simulink model "fusionAlg"  (R2018b)
settings: Solver=FixedStepDiscrete  StartTime=0.0  StopTime=inf  FixedStep=0.01  RelTol=1e-3
PostLoadFcn:
  | if any(exist('dsrtsu_mdlpostloadfcn', 'file') ~= 0), dsrtsu_mdlpostloadfcn('Execute', bdroot); end
model workspace (MAT data in the model file):
  handle : class17 (value not decoded)
(part 2 of 24)

== system fusionAlg/FUSION /FUS_DataAdapter/RadarAdapter/Subsystem15 ==
  <x67_37_Obj_23> : Inport
  Bus Creator : BusCreator  Inputs=2  OutDataTypeStr=Bus: FUS_UINT8_RESERVED_ST
      settings: InheritFromInputs=off
  Bus Creator1 : BusCreator  Inputs=17  OutDataTypeStr=Bus: FUS_RADAR_OBJ_ST  NonVirtualBus=on
      settings: InheritFromInputs=off
  Bus Selector1 : BusSelector  OutputSignals=Obj_ObstacleProb,Obj_XPos_Stdev,Obj_YPos_Stdev,Obj_XVelRel_Stdev,Obj_XAccRel,Obj_ExstProb,Obj_YVelRel,Obj_XVelRel,Obj_XPos,Obj_YPos,Obj_ID,Obj_UpdateFlag,Obj_ValidFlag,Obj_MotionPattern,Obj_Type,Obj_MeasFlag
  Constant : Constant  Value=0  OutDataTypeStr=uint8
  Constant1 : Constant  Value=0  OutDataTypeStr=uint8
  Data Type Conversion : DataTypeConversion  OutDataTypeStr=uint16
  Data Type Conversion{1..5} (5 alike) : DataTypeConversion  OutDataTypeStr=uint8
  <OBJ_23> : Outport
  wires:
  Bus Selector1/10 -> Bus Creator1/10  "<Obj_YPos>"
  Constant1/1 -> Bus Creator/2
  Bus Selector1/8 -> Bus Creator1/8  "<Obj_XVelRel>"
  Bus Selector1/14 -> Data Type Conversion3/1  "<Obj_MotionPattern>"
  Bus Creator1/1 -> <OBJ_23>/1
  Bus Selector1/11 -> Data Type Conversion/1  "<Obj_ID>"
  Bus Selector1/16 -> Data Type Conversion5/1  "<Obj_MeasFlag>"
  Bus Selector1/2 -> Bus Creator1/2  "<Obj_XPos_Stdev>"
  Bus Selector1/6 -> Bus Creator1/6  "<Obj_ExstProb>"
  Bus Selector1/1 -> Bus Creator1/1  "<Obj_ObstacleProb>"
  Bus Selector1/15 -> Data Type Conversion4/1  "<Obj_Type>"
  Constant/1 -> Bus Creator/1
  Bus Selector1/13 -> Data Type Conversion2/1  "<Obj_ValidFlag>"
  Bus Selector1/9 -> Bus Creator1/9  "<Obj_XPos>"
  Bus Selector1/4 -> Bus Creator1/4  "<Obj_XVelRel_Stdev>"
  Bus Selector1/3 -> Bus Creator1/3  "<Obj_YPos_Stdev>"
  Bus Selector1/5 -> Bus Creator1/5  "<Obj_XAccRel>"
  Bus Selector1/7 -> Bus Creator1/7  "<Obj_YVelRel>"
  Bus Selector1/12 -> Data Type Conversion1/1  "<Obj_UpdateFlag>"
  <x67_37_Obj_23>/1 -> Bus Selector1/1
  Bus Creator/1 -> Bus Creator1/17
  Data Type Conversion/1 -> Bus Creator1/11
  Data Type Conversion1/1 -> Bus Creator1/12
  Data Type Conversion2/1 -> Bus Creator1/13
  Data Type Conversion3/1 -> Bus Creator1/14
  Data Type Conversion4/1 -> Bus Creator1/15
  Data Type Conversion5/1 -> Bus Creator1/16

== system fusionAlg/FUSION /FUS_DataAdapter/RadarAdapter/Subsystem16 ==
  <x5E_2E_Obj_14> : Inport
  Bus Creator : BusCreator  Inputs=2  OutDataTypeStr=Bus: FUS_UINT8_RESERVED_ST
      settings: InheritFromInputs=off
  Bus Creator1 : BusCreator  Inputs=17  OutDataTypeStr=Bus: FUS_RADAR_OBJ_ST  NonVirtualBus=on
      settings: InheritFromInputs=off
  Bus Selector1 : BusSelector  OutputSignals=Obj_ObstacleProb,Obj_XPos_Stdev,Obj_YPos_Stdev,Obj_XVelRel_Stdev,Obj_XAccRel,Obj_ExstProb,Obj_YVelRel,Obj_XVelRel,Obj_XPos,Obj_YPos,Obj_ID,Obj_UpdateFlag,Obj_ValidFlag,Obj_MotionPattern,Obj_Type,Obj_MeasFlag
  Constant : Constant  Value=0  OutDataTypeStr=uint8
  Constant1 : Constant  Value=0  OutDataTypeStr=uint8
  Data Type Conversion : DataTypeConversion  OutDataTypeStr=uint16
  Data Type Conversion{1..5} (5 alike) : DataTypeConversion  OutDataTypeStr=uint8
  <OBJ_14> : Outport
  wires:
  Bus Selector1/10 -> Bus Creator1/10  "<Obj_YPos>"
  Constant1/1 -> Bus Creator/2
  Bus Selector1/8 -> Bus Creator1/8  "<Obj_XVelRel>"
  Bus Selector1/14 -> Data Type Conversion3/1  "<Obj_MotionPattern>"
  Bus Creator1/1 -> <OBJ_14>/1
  Bus Selector1/11 -> Data Type Conversion/1  "<Obj_ID>"
  Bus Selector1/16 -> Data Type Conversion5/1  "<Obj_MeasFlag>"
  Bus Selector1/2 -> Bus Creator1/2  "<Obj_XPos_Stdev>"
  Bus Selector1/6 -> Bus Creator1/6  "<Obj_ExstProb>"
  Bus Selector1/1 -> Bus Creator1/1  "<Obj_ObstacleProb>"
  Bus Selector1/15 -> Data Type Conversion4/1  "<Obj_Type>"
  Constant/1 -> Bus Creator/1
  Bus Selector1/13 -> Data Type Conversion2/1  "<Obj_ValidFlag>"
  Bus Selector1/9 -> Bus Creator1/9  "<Obj_XPos>"
  Bus Selector1/4 -> Bus Creator1/4  "<Obj_XVelRel_Stdev>"
  Bus Selector1/3 -> Bus Creator1/3  "<Obj_YPos_Stdev>"
  Bus Selector1/5 -> Bus Creator1/5  "<Obj_XAccRel>"
  Bus Selector1/7 -> Bus Creator1/7  "<Obj_YVelRel>"
  Bus Selector1/12 -> Data Type Conversion1/1  "<Obj_UpdateFlag>"
  <x5E_2E_Obj_14>/1 -> Bus Selector1/1
  Bus Creator/1 -> Bus Creator1/17
  Data Type Conversion/1 -> Bus Creator1/11
  Data Type Conversion1/1 -> Bus Creator1/12
  Data Type Conversion2/1 -> Bus Creator1/13
  Data Type Conversion3/1 -> Bus Creator1/14
  Data Type Conversion4/1 -> Bus Creator1/15
  Data Type Conversion5/1 -> Bus Creator1/16

== system fusionAlg/FUSION /FUS_DataAdapter/RadarAdapter/Subsystem17 ==
  <x5F_2F_Obj_15> : Inport
  Bus Creator : BusCreator  Inputs=2  OutDataTypeStr=Bus: FUS_UINT8_RESERVED_ST
      settings: InheritFromInputs=off
  Bus Creator1 : BusCreator  Inputs=17  OutDataTypeStr=Bus: FUS_RADAR_OBJ_ST  NonVirtualBus=on
      settings: InheritFromInputs=off
  Bus Selector1 : BusSelector  OutputSignals=Obj_ObstacleProb,Obj_XPos_Stdev,Obj_YPos_Stdev,Obj_XVelRel_Stdev,Obj_XAccRel,Obj_ExstProb,Obj_YVelRel,Obj_XVelRel,Obj_XPos,Obj_YPos,Obj_ID,Obj_UpdateFlag,Obj_ValidFlag,Obj_MotionPattern,Obj_Type,Obj_MeasFlag
  Constant : Constant  Value=0  OutDataTypeStr=uint8
  Constant1 : Constant  Value=0  OutDataTypeStr=uint8
  Data Type Conversion : DataTypeConversion  OutDataTypeStr=uint16
  Data Type Conversion{1..5} (5 alike) : DataTypeConversion  OutDataTypeStr=uint8
  <OBJ_15> : Outport
  wires:
  Bus Selector1/10 -> Bus Creator1/10  "<Obj_YPos>"
  Constant1/1 -> Bus Creator/2
  Bus Selector1/8 -> Bus Creator1/8  "<Obj_XVelRel>"
  Bus Selector1/14 -> Data Type Conversion3/1  "<Obj_MotionPattern>"
  Bus Creator1/1 -> <OBJ_15>/1
  Bus Selector1/11 -> Data Type Conversion/1  "<Obj_ID>"
  Bus Selector1/16 -> Data Type Conversion5/1  "<Obj_MeasFlag>"
  Bus Selector1/2 -> Bus Creator1/2  "<Obj_XPos_Stdev>"
  Bus Selector1/6 -> Bus Creator1/6  "<Obj_ExstProb>"
  Bus Selector1/1 -> Bus Creator1/1  "<Obj_ObstacleProb>"
  Bus Selector1/15 -> Data Type Conversion4/1  "<Obj_Type>"
  Constant/1 -> Bus Creator/1
  Bus Selector1/13 -> Data Type Conversion2/1  "<Obj_ValidFlag>"
  Bus Selector1/9 -> Bus Creator1/9  "<Obj_XPos>"
  Bus Selector1/4 -> Bus Creator1/4  "<Obj_XVelRel_Stdev>"
  Bus Selector1/3 -> Bus Creator1/3  "<Obj_YPos_Stdev>"
  Bus Selector1/5 -> Bus Creator1/5  "<Obj_XAccRel>"
  Bus Selector1/7 -> Bus Creator1/7  "<Obj_YVelRel>"
  Bus Selector1/12 -> Data Type Conversion1/1  "<Obj_UpdateFlag>"
  <x5F_2F_Obj_15>/1 -> Bus Selector1/1
  Bus Creator/1 -> Bus Creator1/17
  Data Type Conversion/1 -> Bus Creator1/11
  Data Type Conversion1/1 -> Bus Creator1/12
  Data Type Conversion2/1 -> Bus Creator1/13
  Data Type Conversion3/1 -> Bus Creator1/14
  Data Type Conversion4/1 -> Bus Creator1/15
  Data Type Conversion5/1 -> Bus Creator1/16

== system fusionAlg/FUSION /FUS_DataAdapter/RadarAdapter/Subsystem18 ==
  <x60_30_Obj_16> : Inport
  Bus Creator : BusCreator  Inputs=2  OutDataTypeStr=Bus: FUS_UINT8_RESERVED_ST
      settings: InheritFromInputs=off
  Bus Creator1 : BusCreator  Inputs=17  OutDataTypeStr=Bus: FUS_RADAR_OBJ_ST  NonVirtualBus=on
      settings: InheritFromInputs=off
  Bus Selector1 : BusSelector  OutputSignals=Obj_ObstacleProb,Obj_XPos_Stdev,Obj_YPos_Stdev,Obj_XVelRel_Stdev,Obj_XAccRel,Obj_ExstProb,Obj_YVelRel,Obj_XVelRel,Obj_XPos,Obj_YPos,Obj_ID,Obj_UpdateFlag,Obj_ValidFlag,Obj_MotionPattern,Obj_Type,Obj_MeasFlag
  Constant : Constant  Value=0  OutDataTypeStr=uint8
  Constant1 : Constant  Value=0  OutDataTypeStr=uint8
  Data Type Conversion : DataTypeConversion  OutDataTypeStr=uint16
  Data Type Conversion{1..5} (5 alike) : DataTypeConversion  OutDataTypeStr=uint8
  <OBJ_16> : Outport
  wires:
  Bus Selector1/10 -> Bus Creator1/10  "<Obj_YPos>"
  Constant1/1 -> Bus Creator/2
  Bus Selector1/8 -> Bus Creator1/8  "<Obj_XVelRel>"
  Bus Selector1/14 -> Data Type Conversion3/1  "<Obj_MotionPattern>"
  Bus Creator1/1 -> <OBJ_16>/1
  Bus Selector1/11 -> Data Type Conversion/1  "<Obj_ID>"
  Bus Selector1/16 -> Data Type Conversion5/1  "<Obj_MeasFlag>"
  Bus Selector1/2 -> Bus Creator1/2  "<Obj_XPos_Stdev>"
  Bus Selector1/6 -> Bus Creator1/6  "<Obj_ExstProb>"
  Bus Selector1/1 -> Bus Creator1/1  "<Obj_ObstacleProb>"
  Bus Selector1/15 -> Data Type Conversion4/1  "<Obj_Type>"
  Constant/1 -> Bus Creator/1
  Bus Selector1/13 -> Data Type Conversion2/1  "<Obj_ValidFlag>"
  Bus Selector1/9 -> Bus Creator1/9  "<Obj_XPos>"
  Bus Selector1/4 -> Bus Creator1/4  "<Obj_XVelRel_Stdev>"
  Bus Selector1/3 -> Bus Creator1/3  "<Obj_YPos_Stdev>"
  Bus Selector1/5 -> Bus Creator1/5  "<Obj_XAccRel>"
  Bus Selector1/7 -> Bus Creator1/7  "<Obj_YVelRel>"
  Bus Selector1/12 -> Data Type Conversion1/1  "<Obj_UpdateFlag>"
  <x60_30_Obj_16>/1 -> Bus Selector1/1
  Bus Creator/1 -> Bus Creator1/17
  Data Type Conversion/1 -> Bus Creator1/11
  Data Type Conversion1/1 -> Bus Creator1/12
  Data Type Conversion2/1 -> Bus Creator1/13
  Data Type Conversion3/1 -> Bus Creator1/14
  Data Type Conversion4/1 -> Bus Creator1/15
  Data Type Conversion5/1 -> Bus Creator1/16

== system fusionAlg/FUSION /FUS_DataAdapter/RadarAdapter/Subsystem19 ==
  <x61_31_Obj_17> : Inport
  Bus Creator : BusCreator  Inputs=2  OutDataTypeStr=Bus: FUS_UINT8_RESERVED_ST
      settings: InheritFromInputs=off
  Bus Creator1 : BusCreator  Inputs=17  OutDataTypeStr=Bus: FUS_RADAR_OBJ_ST  NonVirtualBus=on
      settings: InheritFromInputs=off
  Bus Selector1 : BusSelector  OutputSignals=Obj_ObstacleProb,Obj_XPos_Stdev,Obj_YPos_Stdev,Obj_XVelRel_Stdev,Obj_XAccRel,Obj_ExstProb,Obj_YVelRel,Obj_XVelRel,Obj_XPos,Obj_YPos,Obj_ID,Obj_UpdateFlag,Obj_ValidFlag,Obj_MotionPattern,Obj_Type,Obj_MeasFlag
  Constant : Constant  Value=0  OutDataTypeStr=uint8
  Constant1 : Constant  Value=0  OutDataTypeStr=uint8
  Data Type Conversion : DataTypeConversion  OutDataTypeStr=uint16
  Data Type Conversion{1..5} (5 alike) : DataTypeConversion  OutDataTypeStr=uint8
  <OBJ_17> : Outport
  wires:
  Bus Selector1/10 -> Bus Creator1/10  "<Obj_YPos>"
  Constant1/1 -> Bus Creator/2
  Bus Selector1/8 -> Bus Creator1/8  "<Obj_XVelRel>"
  Bus Selector1/14 -> Data Type Conversion3/1  "<Obj_MotionPattern>"
  Bus Creator1/1 -> <OBJ_17>/1
  Bus Selector1/11 -> Data Type Conversion/1  "<Obj_ID>"
  Bus Selector1/16 -> Data Type Conversion5/1  "<Obj_MeasFlag>"
  Bus Selector1/2 -> Bus Creator1/2  "<Obj_XPos_Stdev>"
  Bus Selector1/6 -> Bus Creator1/6  "<Obj_ExstProb>"
  Bus Selector1/1 -> Bus Creator1/1  "<Obj_ObstacleProb>"
  Bus Selector1/15 -> Data Type Conversion4/1  "<Obj_Type>"
  Constant/1 -> Bus Creator/1
  Bus Selector1/13 -> Data Type Conversion2/1  "<Obj_ValidFlag>"
  Bus Selector1/9 -> Bus Creator1/9  "<Obj_XPos>"
  Bus Selector1/4 -> Bus Creator1/4  "<Obj_XVelRel_Stdev>"
  Bus Selector1/3 -> Bus Creator1/3  "<Obj_YPos_Stdev>"
  Bus Selector1/5 -> Bus Creator1/5  "<Obj_XAccRel>"
  Bus Selector1/7 -> Bus Creator1/7  "<Obj_YVelRel>"
  Bus Selector1/12 -> Data Type Conversion1/1  "<Obj_UpdateFlag>"
  <x61_31_Obj_17>/1 -> Bus Selector1/1
  Bus Creator/1 -> Bus Creator1/17
  Data Type Conversion/1 -> Bus Creator1/11
  Data Type Conversion1/1 -> Bus Creator1/12
  Data Type Conversion2/1 -> Bus Creator1/13
  Data Type Conversion3/1 -> Bus Creator1/14
  Data Type Conversion4/1 -> Bus Creator1/15
  Data Type Conversion5/1 -> Bus Creator1/16

== system fusionAlg/FUSION /FUS_DataAdapter/RadarAdapter/Subsystem2 ==
  <x52_22_Obj_02> : Inport
  Bus Creator : BusCreator  Inputs=2  OutDataTypeStr=Bus: FUS_UINT8_RESERVED_ST
      settings: InheritFromInputs=off
  Bus Creator1 : BusCreator  Inputs=17  OutDataTypeStr=Bus: FUS_RADAR_OBJ_ST  NonVirtualBus=on
      settings: InheritFromInputs=off
  Bus Selector1 : BusSelector  OutputSignals=Obj_ObstacleProb,Obj_XPos_Stdev,Obj_YPos_Stdev,Obj_XVelRel_Stdev,Obj_XAccRel,Obj_ExstProb,Obj_YVelRel,Obj_XVelRel,Obj_XPos,Obj_YPos,Obj_ID,Obj_UpdateFlag,Obj_ValidFlag,Obj_MotionPattern,Obj_Type,Obj_MeasFlag
  Constant : Constant  Value=0  OutDataTypeStr=uint8
  Constant1 : Constant  Value=0  OutDataTypeStr=uint8
  Data Type Conversion : DataTypeConversion  OutDataTypeStr=uint16
  Data Type Conversion{1..5} (5 alike) : DataTypeConversion  OutDataTypeStr=uint8
  <OBJ_02> : Outport
  wires:
  Bus Selector1/10 -> Bus Creator1/10  "<Obj_YPos>"
  Constant1/1 -> Bus Creator/2
  Bus Selector1/8 -> Bus Creator1/8  "<Obj_XVelRel>"
  Bus Selector1/14 -> Data Type Conversion3/1  "<Obj_MotionPattern>"
  Bus Creator1/1 -> <OBJ_02>/1
  Bus Selector1/11 -> Data Type Conversion/1  "<Obj_ID>"
  Bus Selector1/16 -> Data Type Conversion5/1  "<Obj_MeasFlag>"
  Bus Selector1/2 -> Bus Creator1/2  "<Obj_XPos_Stdev>"
  Bus Selector1/6 -> Bus Creator1/6  "<Obj_ExstProb>"
  Bus Selector1/1 -> Bus Creator1/1  "<Obj_ObstacleProb>"
  Bus Selector1/15 -> Data Type Conversion4/1  "<Obj_Type>"
  Constant/1 -> Bus Creator/1
  Bus Selector1/13 -> Data Type Conversion2/1  "<Obj_ValidFlag>"
  Bus Selector1/9 -> Bus Creator1/9  "<Obj_XPos>"
  Bus Selector1/4 -> Bus Creator1/4  "<Obj_XVelRel_Stdev>"
  Bus Selector1/3 -> Bus Creator1/3  "<Obj_YPos_Stdev>"
  Bus Selector1/5 -> Bus Creator1/5  "<Obj_XAccRel>"
  Bus Selector1/7 -> Bus Creator1/7  "<Obj_YVelRel>"
  Bus Selector1/12 -> Data Type Conversion1/1  "<Obj_UpdateFlag>"
  <x52_22_Obj_02>/1 -> Bus Selector1/1
  Bus Creator/1 -> Bus Creator1/17
  Data Type Conversion/1 -> Bus Creator1/11
  Data Type Conversion1/1 -> Bus Creator1/12
  Data Type Conversion2/1 -> Bus Creator1/13
  Data Type Conversion3/1 -> Bus Creator1/14
  Data Type Conversion4/1 -> Bus Creator1/15
  Data Type Conversion5/1 -> Bus Creator1/16

== system fusionAlg/FUSION /FUS_DataAdapter/RadarAdapter/Subsystem20 ==
  <x62_32_Obj_18> : Inport
  Bus Creator : BusCreator  Inputs=2  OutDataTypeStr=Bus: FUS_UINT8_RESERVED_ST
      settings: InheritFromInputs=off
  Bus Creator1 : BusCreator  Inputs=17  OutDataTypeStr=Bus: FUS_RADAR_OBJ_ST  NonVirtualBus=on
      settings: InheritFromInputs=off
  Bus Selector1 : BusSelector  OutputSignals=Obj_ObstacleProb,Obj_XPos_Stdev,Obj_YPos_Stdev,Obj_XVelRel_Stdev,Obj_XAccRel,Obj_ExstProb,Obj_YVelRel,Obj_XVelRel,Obj_XPos,Obj_YPos,Obj_ID,Obj_UpdateFlag,Obj_ValidFlag,Obj_MotionPattern,Obj_Type,Obj_MeasFlag
  Constant : Constant  Value=0  OutDataTypeStr=uint8
  Constant1 : Constant  Value=0  OutDataTypeStr=uint8
  Data Type Conversion : DataTypeConversion  OutDataTypeStr=uint16
  Data Type Conversion{1..5} (5 alike) : DataTypeConversion  OutDataTypeStr=uint8
  <OBJ_18> : Outport
  wires:
  Bus Selector1/10 -> Bus Creator1/10  "<Obj_YPos>"
  Constant1/1 -> Bus Creator/2
  Bus Selector1/8 -> Bus Creator1/8  "<Obj_XVelRel>"
  Bus Selector1/14 -> Data Type Conversion3/1  "<Obj_MotionPattern>"
  Bus Creator1/1 -> <OBJ_18>/1
  Bus Selector1/11 -> Data Type Conversion/1  "<Obj_ID>"
  Bus Selector1/16 -> Data Type Conversion5/1  "<Obj_MeasFlag>"
  Bus Selector1/2 -> Bus Creator1/2  "<Obj_XPos_Stdev>"
  Bus Selector1/6 -> Bus Creator1/6  "<Obj_ExstProb>"
  Bus Selector1/1 -> Bus Creator1/1  "<Obj_ObstacleProb>"
  Bus Selector1/15 -> Data Type Conversion4/1  "<Obj_Type>"
  Constant/1 -> Bus Creator/1
  Bus Selector1/13 -> Data Type Conversion2/1  "<Obj_ValidFlag>"
  Bus Selector1/9 -> Bus Creator1/9  "<Obj_XPos>"
  Bus Selector1/4 -> Bus Creator1/4  "<Obj_XVelRel_Stdev>"
  Bus Selector1/3 -> Bus Creator1/3  "<Obj_YPos_Stdev>"
  Bus Selector1/5 -> Bus Creator1/5  "<Obj_XAccRel>"
  Bus Selector1/7 -> Bus Creator1/7  "<Obj_YVelRel>"
  Bus Selector1/12 -> Data Type Conversion1/1  "<Obj_UpdateFlag>"
  <x62_32_Obj_18>/1 -> Bus Selector1/1
  Bus Creator/1 -> Bus Creator1/17
  Data Type Conversion/1 -> Bus Creator1/11
  Data Type Conversion1/1 -> Bus Creator1/12
  Data Type Conversion2/1 -> Bus Creator1/13
  Data Type Conversion3/1 -> Bus Creator1/14
  Data Type Conversion4/1 -> Bus Creator1/15
  Data Type Conversion5/1 -> Bus Creator1/16

== system fusionAlg/FUSION /FUS_DataAdapter/RadarAdapter/Subsystem21 ==
  <x63_33_Obj_19> : Inport
  Bus Creator : BusCreator  Inputs=2  OutDataTypeStr=Bus: FUS_UINT8_RESERVED_ST
      settings: InheritFromInputs=off
  Bus Creator1 : BusCreator  Inputs=17  OutDataTypeStr=Bus: FUS_RADAR_OBJ_ST  NonVirtualBus=on
      settings: InheritFromInputs=off
  Bus Selector1 : BusSelector  OutputSignals=Obj_ObstacleProb,Obj_XPos_Stdev,Obj_YPos_Stdev,Obj_XVelRel_Stdev,Obj_XAccRel,Obj_ExstProb,Obj_YVelRel,Obj_XVelRel,Obj_XPos,Obj_YPos,Obj_ID,Obj_UpdateFlag,Obj_ValidFlag,Obj_MotionPattern,Obj_Type,Obj_MeasFlag
  Constant : Constant  Value=0  OutDataTypeStr=uint8
  Constant1 : Constant  Value=0  OutDataTypeStr=uint8
  Data Type Conversion : DataTypeConversion  OutDataTypeStr=uint16
  Data Type Conversion{1..5} (5 alike) : DataTypeConversion  OutDataTypeStr=uint8
  <OBJ_19> : Outport
  wires:
  Bus Selector1/10 -> Bus Creator1/10  "<Obj_YPos>"
  Constant1/1 -> Bus Creator/2
  Bus Selector1/8 -> Bus Creator1/8  "<Obj_XVelRel>"
  Bus Selector1/14 -> Data Type Conversion3/1  "<Obj_MotionPattern>"
  Bus Creator1/1 -> <OBJ_19>/1
  Bus Selector1/11 -> Data Type Conversion/1  "<Obj_ID>"
  Bus Selector1/16 -> Data Type Conversion5/1  "<Obj_MeasFlag>"
  Bus Selector1/2 -> Bus Creator1/2  "<Obj_XPos_Stdev>"
  Bus Selector1/6 -> Bus Creator1/6  "<Obj_ExstProb>"
  Bus Selector1/1 -> Bus Creator1/1  "<Obj_ObstacleProb>"
  Bus Selector1/15 -> Data Type Conversion4/1  "<Obj_Type>"
  Constant/1 -> Bus Creator/1
  Bus Selector1/13 -> Data Type Conversion2/1  "<Obj_ValidFlag>"
  Bus Selector1/9 -> Bus Creator1/9  "<Obj_XPos>"
  Bus Selector1/4 -> Bus Creator1/4  "<Obj_XVelRel_Stdev>"
  Bus Selector1/3 -> Bus Creator1/3  "<Obj_YPos_Stdev>"
  Bus Selector1/5 -> Bus Creator1/5  "<Obj_XAccRel>"
  Bus Selector1/7 -> Bus Creator1/7  "<Obj_YVelRel>"
  Bus Selector1/12 -> Data Type Conversion1/1  "<Obj_UpdateFlag>"
  <x63_33_Obj_19>/1 -> Bus Selector1/1
  Bus Creator/1 -> Bus Creator1/17
  Data Type Conversion/1 -> Bus Creator1/11
  Data Type Conversion1/1 -> Bus Creator1/12
  Data Type Conversion2/1 -> Bus Creator1/13
  Data Type Conversion3/1 -> Bus Creator1/14
  Data Type Conversion4/1 -> Bus Creator1/15
  Data Type Conversion5/1 -> Bus Creator1/16

== system fusionAlg/FUSION /FUS_DataAdapter/RadarAdapter/Subsystem22 ==
  <x64_34_Obj_20> : Inport
  Bus Creator : BusCreator  Inputs=2  OutDataTypeStr=Bus: FUS_UINT8_RESERVED_ST
      settings: InheritFromInputs=off
  Bus Creator1 : BusCreator  Inputs=17  OutDataTypeStr=Bus: FUS_RADAR_OBJ_ST  NonVirtualBus=on
      settings: InheritFromInputs=off
  Bus Selector1 : BusSelector  OutputSignals=Obj_ObstacleProb,Obj_XPos_Stdev,Obj_YPos_Stdev,Obj_XVelRel_Stdev,Obj_XAccRel,Obj_ExstProb,Obj_YVelRel,Obj_XVelRel,Obj_XPos,Obj_YPos,Obj_ID,Obj_UpdateFlag,Obj_ValidFlag,Obj_MotionPattern,Obj_Type,Obj_MeasFlag
  Constant : Constant  Value=0  OutDataTypeStr=uint8
  Constant1 : Constant  Value=0  OutDataTypeStr=uint8
  Data Type Conversion : DataTypeConversion  OutDataTypeStr=uint16
  Data Type Conversion{1..5} (5 alike) : DataTypeConversion  OutDataTypeStr=uint8
  <OBJ_20> : Outport
  wires:
  Bus Selector1/10 -> Bus Creator1/10  "<Obj_YPos>"
  Constant1/1 -> Bus Creator/2
  Bus Selector1/8 -> Bus Creator1/8  "<Obj_XVelRel>"
  Bus Selector1/14 -> Data Type Conversion3/1  "<Obj_MotionPattern>"
  Bus Creator1/1 -> <OBJ_20>/1
  Bus Selector1/11 -> Data Type Conversion/1  "<Obj_ID>"
  Bus Selector1/16 -> Data Type Conversion5/1  "<Obj_MeasFlag>"
  Bus Selector1/2 -> Bus Creator1/2  "<Obj_XPos_Stdev>"
  Bus Selector1/6 -> Bus Creator1/6  "<Obj_ExstProb>"
  Bus Selector1/1 -> Bus Creator1/1  "<Obj_ObstacleProb>"
  Bus Selector1/15 -> Data Type Conversion4/1  "<Obj_Type>"
  Constant/1 -> Bus Creator/1
  Bus Selector1/13 -> Data Type Conversion2/1  "<Obj_ValidFlag>"
  Bus Selector1/9 -> Bus Creator1/9  "<Obj_XPos>"
  Bus Selector1/4 -> Bus Creator1/4  "<Obj_XVelRel_Stdev>"
  Bus Selector1/3 -> Bus Creator1/3  "<Obj_YPos_Stdev>"
  Bus Selector1/5 -> Bus Creator1/5  "<Obj_XAccRel>"
  Bus Selector1/7 -> Bus Creator1/7  "<Obj_YVelRel>"
  Bus Selector1/12 -> Data Type Conversion1/1  "<Obj_UpdateFlag>"
  <x64_34_Obj_20>/1 -> Bus Selector1/1
  Bus Creator/1 -> Bus Creator1/17
  Data Type Conversion/1 -> Bus Creator1/11
  Data Type Conversion1/1 -> Bus Creator1/12
  Data Type Conversion2/1 -> Bus Creator1/13
  Data Type Conversion3/1 -> Bus Creator1/14
  Data Type Conversion4/1 -> Bus Creator1/15
  Data Type Conversion5/1 -> Bus Creator1/16

== system fusionAlg/FUSION /FUS_DataAdapter/RadarAdapter/Subsystem23 ==
  <x65_35_Obj_21> : Inport
  Bus Creator : BusCreator  Inputs=2  OutDataTypeStr=Bus: FUS_UINT8_RESERVED_ST
      settings: InheritFromInputs=off
  Bus Creator1 : BusCreator  Inputs=17  OutDataTypeStr=Bus: FUS_RADAR_OBJ_ST  NonVirtualBus=on
      settings: InheritFromInputs=off
  Bus Selector1 : BusSelector  OutputSignals=Obj_ObstacleProb,Obj_XPos_Stdev,Obj_YPos_Stdev,Obj_XVelRel_Stdev,Obj_XAccRel,Obj_ExstProb,Obj_YVelRel,Obj_XVelRel,Obj_XPos,Obj_YPos,Obj_ID,Obj_UpdateFlag,Obj_ValidFlag,Obj_MotionPattern,Obj_Type,Obj_MeasFlag
  Constant : Constant  Value=0  OutDataTypeStr=uint8
  Constant1 : Constant  Value=0  OutDataTypeStr=uint8
  Data Type Conversion : DataTypeConversion  OutDataTypeStr=uint16
  Data Type Conversion{1..5} (5 alike) : DataTypeConversion  OutDataTypeStr=uint8
  <OBJ_21> : Outport
  wires:
  Bus Selector1/10 -> Bus Creator1/10  "<Obj_YPos>"
  Constant1/1 -> Bus Creator/2
  Bus Selector1/8 -> Bus Creator1/8  "<Obj_XVelRel>"
  Bus Selector1/14 -> Data Type Conversion3/1  "<Obj_MotionPattern>"
  Bus Creator1/1 -> <OBJ_21>/1
  Bus Selector1/11 -> Data Type Conversion/1  "<Obj_ID>"
  Bus Selector1/16 -> Data Type Conversion5/1  "<Obj_MeasFlag>"
  Bus Selector1/2 -> Bus Creator1/2  "<Obj_XPos_Stdev>"
  Bus Selector1/6 -> Bus Creator1/6  "<Obj_ExstProb>"
  Bus Selector1/1 -> Bus Creator1/1  "<Obj_ObstacleProb>"
  Bus Selector1/15 -> Data Type Conversion4/1  "<Obj_Type>"
  Constant/1 -> Bus Creator/1
  Bus Selector1/13 -> Data Type Conversion2/1  "<Obj_ValidFlag>"
  Bus Selector1/9 -> Bus Creator1/9  "<Obj_XPos>"
  Bus Selector1/4 -> Bus Creator1/4  "<Obj_XVelRel_Stdev>"
  Bus Selector1/3 -> Bus Creator1/3  "<Obj_YPos_Stdev>"
  Bus Selector1/5 -> Bus Creator1/5  "<Obj_XAccRel>"
  Bus Selector1/7 -> Bus Creator1/7  "<Obj_YVelRel>"
  Bus Selector1/12 -> Data Type Conversion1/1  "<Obj_UpdateFlag>"
  <x65_35_Obj_21>/1 -> Bus Selector1/1
  Bus Creator/1 -> Bus Creator1/17
  Data Type Conversion/1 -> Bus Creator1/11
  Data Type Conversion1/1 -> Bus Creator1/12
  Data Type Conversion2/1 -> Bus Creator1/13
  Data Type Conversion3/1 -> Bus Creator1/14
  Data Type Conversion4/1 -> Bus Creator1/15
  Data Type Conversion5/1 -> Bus Creator1/16

== system fusionAlg/FUSION /FUS_DataAdapter/RadarAdapter/Subsystem24 ==
  <x68_38_Obj_24> : Inport
  Bus Creator : BusCreator  Inputs=2  OutDataTypeStr=Bus: FUS_UINT8_RESERVED_ST
      settings: InheritFromInputs=off
  Bus Creator1 : BusCreator  Inputs=17  OutDataTypeStr=Bus: FUS_RADAR_OBJ_ST  NonVirtualBus=on
      settings: InheritFromInputs=off
  Bus Selector1 : BusSelector  OutputSignals=Obj_ObstacleProb,Obj_XPos_Stdev,Obj_YPos_Stdev,Obj_XVelRel_Stdev,Obj_XAccRel,Obj_ExstProb,Obj_YVelRel,Obj_XVelRel,Obj_XPos,Obj_YPos,Obj_ID,Obj_UpdateFlag,Obj_ValidFlag,Obj_MotionPattern,Obj_Type,Obj_MeasFlag
  Constant : Constant  Value=0  OutDataTypeStr=uint8
  Constant1 : Constant  Value=0  OutDataTypeStr=uint8
  Data Type Conversion : DataTypeConversion  OutDataTypeStr=uint16
  Data Type Conversion{1..5} (5 alike) : DataTypeConversion  OutDataTypeStr=uint8
  <OBJ_24> : Outport
  wires:
  Bus Selector1/10 -> Bus Creator1/10  "<Obj_YPos>"
  Constant1/1 -> Bus Creator/2
  Bus Selector1/8 -> Bus Creator1/8  "<Obj_XVelRel>"
  Bus Selector1/14 -> Data Type Conversion3/1  "<Obj_MotionPattern>"
  Bus Creator1/1 -> <OBJ_24>/1
  Bus Selector1/11 -> Data Type Conversion/1  "<Obj_ID>"
  Bus Selector1/16 -> Data Type Conversion5/1  "<Obj_MeasFlag>"
  Bus Selector1/2 -> Bus Creator1/2  "<Obj_XPos_Stdev>"
  Bus Selector1/6 -> Bus Creator1/6  "<Obj_ExstProb>"
  Bus Selector1/1 -> Bus Creator1/1  "<Obj_ObstacleProb>"
  Bus Selector1/15 -> Data Type Conversion4/1  "<Obj_Type>"
  Constant/1 -> Bus Creator/1
  Bus Selector1/13 -> Data Type Conversion2/1  "<Obj_ValidFlag>"
  Bus Selector1/9 -> Bus Creator1/9  "<Obj_XPos>"
  Bus Selector1/4 -> Bus Creator1/4  "<Obj_XVelRel_Stdev>"
  Bus Selector1/3 -> Bus Creator1/3  "<Obj_YPos_Stdev>"
  Bus Selector1/5 -> Bus Creator1/5  "<Obj_XAccRel>"
  Bus Selector1/7 -> Bus Creator1/7  "<Obj_YVelRel>"
  Bus Selector1/12 -> Data Type Conversion1/1  "<Obj_UpdateFlag>"
  <x68_38_Obj_24>/1 -> Bus Selector1/1
  Bus Creator/1 -> Bus Creator1/17
  Data Type Conversion/1 -> Bus Creator1/11
  Data Type Conversion1/1 -> Bus Creator1/12
  Data Type Conversion2/1 -> Bus Creator1/13
  Data Type Conversion3/1 -> Bus Creator1/14
  Data Type Conversion4/1 -> Bus Creator1/15
  Data Type Conversion5/1 -> Bus Creator1/16

== system fusionAlg/FUSION /FUS_DataAdapter/RadarAdapter/Subsystem25 ==
  <x69_39_Obj_25> : Inport
  Bus Creator : BusCreator  Inputs=2  OutDataTypeStr=Bus: FUS_UINT8_RESERVED_ST
      settings: InheritFromInputs=off
  Bus Creator1 : BusCreator  Inputs=17  OutDataTypeStr=Bus: FUS_RADAR_OBJ_ST  NonVirtualBus=on
      settings: InheritFromInputs=off
  Bus Selector1 : BusSelector  OutputSignals=Obj_ObstacleProb,Obj_XPos_Stdev,Obj_YPos_Stdev,Obj_XVelRel_Stdev,Obj_XAccRel,Obj_ExstProb,Obj_YVelRel,Obj_XVelRel,Obj_XPos,Obj_YPos,Obj_ID,Obj_UpdateFlag,Obj_ValidFlag,Obj_MotionPattern,Obj_Type,Obj_MeasFlag
  Constant : Constant  Value=0  OutDataTypeStr=uint8
  Constant1 : Constant  Value=0  OutDataTypeStr=uint8
  Data Type Conversion : DataTypeConversion  OutDataTypeStr=uint16
  Data Type Conversion{1..5} (5 alike) : DataTypeConversion  OutDataTypeStr=uint8
  <OBJ_25> : Outport
  wires:
  Bus Selector1/10 -> Bus Creator1/10  "<Obj_YPos>"
  Constant1/1 -> Bus Creator/2
  Bus Selector1/8 -> Bus Creator1/8  "<Obj_XVelRel>"
  Bus Selector1/14 -> Data Type Conversion3/1  "<Obj_MotionPattern>"
  Bus Creator1/1 -> <OBJ_25>/1
  Bus Selector1/11 -> Data Type Conversion/1  "<Obj_ID>"
  Bus Selector1/16 -> Data Type Conversion5/1  "<Obj_MeasFlag>"
  Bus Selector1/2 -> Bus Creator1/2  "<Obj_XPos_Stdev>"
  Bus Selector1/6 -> Bus Creator1/6  "<Obj_ExstProb>"
  Bus Selector1/1 -> Bus Creator1/1  "<Obj_ObstacleProb>"
  Bus Selector1/15 -> Data Type Conversion4/1  "<Obj_Type>"
  Constant/1 -> Bus Creator/1
  Bus Selector1/13 -> Data Type Conversion2/1  "<Obj_ValidFlag>"
  Bus Selector1/9 -> Bus Creator1/9  "<Obj_XPos>"
  Bus Selector1/4 -> Bus Creator1/4  "<Obj_XVelRel_Stdev>"
  Bus Selector1/3 -> Bus Creator1/3  "<Obj_YPos_Stdev>"
  Bus Selector1/5 -> Bus Creator1/5  "<Obj_XAccRel>"
  Bus Selector1/7 -> Bus Creator1/7  "<Obj_YVelRel>"
  Bus Selector1/12 -> Data Type Conversion1/1  "<Obj_UpdateFlag>"
  <x69_39_Obj_25>/1 -> Bus Selector1/1
  Bus Creator/1 -> Bus Creator1/17
  Data Type Conversion/1 -> Bus Creator1/11
  Data Type Conversion1/1 -> Bus Creator1/12
  Data Type Conversion2/1 -> Bus Creator1/13
  Data Type Conversion3/1 -> Bus Creator1/14
  Data Type Conversion4/1 -> Bus Creator1/15
  Data Type Conversion5/1 -> Bus Creator1/16

== system fusionAlg/FUSION /FUS_DataAdapter/RadarAdapter/Subsystem26 ==
  <x72_42_Obj_34> : Inport
  Bus Creator : BusCreator  Inputs=2  OutDataTypeStr=Bus: FUS_UINT8_RESERVED_ST
      settings: InheritFromInputs=off
  Bus Creator1 : BusCreator  Inputs=17  OutDataTypeStr=Bus: FUS_RADAR_OBJ_ST  NonVirtualBus=on
      settings: InheritFromInputs=off
  Bus Selector1 : BusSelector  OutputSignals=Obj_ObstacleProb,Obj_XPos_Stdev,Obj_YPos_Stdev,Obj_XVelRel_Stdev,Obj_XAccRel,Obj_ExstProb,Obj_YVelRel,Obj_XVelRel,Obj_XPos,Obj_YPos,Obj_ID,Obj_UpdateFlag,Obj_ValidFlag,Obj_MotionPattern,Obj_Type,Obj_MeasFlag
  Constant : Constant  Value=0  OutDataTypeStr=uint8
  Constant1 : Constant  Value=0  OutDataTypeStr=uint8
  Data Type Conversion : DataTypeConversion  OutDataTypeStr=uint16
  Data Type Conversion{1..5} (5 alike) : DataTypeConversion  OutDataTypeStr=uint8
  <OBJ_34> : Outport
  wires:
  Bus Selector1/10 -> Bus Creator1/10  "<Obj_YPos>"
  Constant1/1 -> Bus Creator/2
  Bus Selector1/8 -> Bus Creator1/8  "<Obj_XVelRel>"
  Bus Selector1/14 -> Data Type Conversion3/1  "<Obj_MotionPattern>"
  Bus Creator1/1 -> <OBJ_34>/1
  Bus Selector1/11 -> Data Type Conversion/1  "<Obj_ID>"
  Bus Selector1/16 -> Data Type Conversion5/1  "<Obj_MeasFlag>"
  Bus Selector1/2 -> Bus Creator1/2  "<Obj_XPos_Stdev>"
  Bus Selector1/6 -> Bus Creator1/6  "<Obj_ExstProb>"
  Bus Selector1/1 -> Bus Creator1/1  "<Obj_ObstacleProb>"
  Bus Selector1/15 -> Data Type Conversion4/1  "<Obj_Type>"
  Constant/1 -> Bus Creator/1
  Bus Selector1/13 -> Data Type Conversion2/1  "<Obj_ValidFlag>"
  Bus Selector1/9 -> Bus Creator1/9  "<Obj_XPos>"
  Bus Selector1/4 -> Bus Creator1/4  "<Obj_XVelRel_Stdev>"
  Bus Selector1/3 -> Bus Creator1/3  "<Obj_YPos_Stdev>"
  Bus Selector1/5 -> Bus Creator1/5  "<Obj_XAccRel>"
  Bus Selector1/7 -> Bus Creator1/7  "<Obj_YVelRel>"
  Bus Selector1/12 -> Data Type Conversion1/1  "<Obj_UpdateFlag>"
  <x72_42_Obj_34>/1 -> Bus Selector1/1
  Bus Creator/1 -> Bus Creator1/17
  Data Type Conversion/1 -> Bus Creator1/11
  Data Type Conversion1/1 -> Bus Creator1/12
  Data Type Conversion2/1 -> Bus Creator1/13
  Data Type Conversion3/1 -> Bus Creator1/14
  Data Type Conversion4/1 -> Bus Creator1/15
  Data Type Conversion5/1 -> Bus Creator1/16

== system fusionAlg/FUSION /FUS_DataAdapter/RadarAdapter/Subsystem27 ==
  <x73_43_Obj_35> : Inport
  Bus Creator : BusCreator  Inputs=2  OutDataTypeStr=Bus: FUS_UINT8_RESERVED_ST
      settings: InheritFromInputs=off
  Bus Creator1 : BusCreator  Inputs=17  OutDataTypeStr=Bus: FUS_RADAR_OBJ_ST  NonVirtualBus=on
      settings: InheritFromInputs=off
  Bus Selector1 : BusSelector  OutputSignals=Obj_ObstacleProb,Obj_XPos_Stdev,Obj_YPos_Stdev,Obj_XVelRel_Stdev,Obj_XAccRel,Obj_ExstProb,Obj_YVelRel,Obj_XVelRel,Obj_XPos,Obj_YPos,Obj_ID,Obj_UpdateFlag,Obj_ValidFlag,Obj_MotionPattern,Obj_Type,Obj_MeasFlag
  Constant : Constant  Value=0  OutDataTypeStr=uint8
  Constant1 : Constant  Value=0  OutDataTypeStr=uint8
  Data Type Conversion : DataTypeConversion  OutDataTypeStr=uint16
  Data Type Conversion{1..5} (5 alike) : DataTypeConversion  OutDataTypeStr=uint8
  <OBJ_35> : Outport
  wires:
  Bus Selector1/10 -> Bus Creator1/10  "<Obj_YPos>"
  Constant1/1 -> Bus Creator/2
  Bus Selector1/8 -> Bus Creator1/8  "<Obj_XVelRel>"
  Bus Selector1/14 -> Data Type Conversion3/1  "<Obj_MotionPattern>"
  Bus Creator1/1 -> <OBJ_35>/1
  Bus Selector1/11 -> Data Type Conversion/1  "<Obj_ID>"
  Bus Selector1/16 -> Data Type Conversion5/1  "<Obj_MeasFlag>"
  Bus Selector1/2 -> Bus Creator1/2  "<Obj_XPos_Stdev>"
  Bus Selector1/6 -> Bus Creator1/6  "<Obj_ExstProb>"
  Bus Selector1/1 -> Bus Creator1/1  "<Obj_ObstacleProb>"
  Bus Selector1/15 -> Data Type Conversion4/1  "<Obj_Type>"
  Constant/1 -> Bus Creator/1
  Bus Selector1/13 -> Data Type Conversion2/1  "<Obj_ValidFlag>"
  Bus Selector1/9 -> Bus Creator1/9  "<Obj_XPos>"
  Bus Selector1/4 -> Bus Creator1/4  "<Obj_XVelRel_Stdev>"
  Bus Selector1/3 -> Bus Creator1/3  "<Obj_YPos_Stdev>"
  Bus Selector1/5 -> Bus Creator1/5  "<Obj_XAccRel>"
  Bus Selector1/7 -> Bus Creator1/7  "<Obj_YVelRel>"
  Bus Selector1/12 -> Data Type Conversion1/1  "<Obj_UpdateFlag>"
  <x73_43_Obj_35>/1 -> Bus Selector1/1
  Bus Creator/1 -> Bus Creator1/17
  Data Type Conversion/1 -> Bus Creator1/11
  Data Type Conversion1/1 -> Bus Creator1/12
  Data Type Conversion2/1 -> Bus Creator1/13
  Data Type Conversion3/1 -> Bus Creator1/14
  Data Type Conversion4/1 -> Bus Creator1/15
  Data Type Conversion5/1 -> Bus Creator1/16

== system fusionAlg/FUSION /FUS_DataAdapter/RadarAdapter/Subsystem28 ==
  <x74_44_Obj_36> : Inport
  Bus Creator : BusCreator  Inputs=2  OutDataTypeStr=Bus: FUS_UINT8_RESERVED_ST
      settings: InheritFromInputs=off
  Bus Creator1 : BusCreator  Inputs=17  OutDataTypeStr=Bus: FUS_RADAR_OBJ_ST  NonVirtualBus=on
      settings: InheritFromInputs=off
  Bus Selector1 : BusSelector  OutputSignals=Obj_ObstacleProb,Obj_XPos_Stdev,Obj_YPos_Stdev,Obj_XVelRel_Stdev,Obj_XAccRel,Obj_ExstProb,Obj_YVelRel,Obj_XVelRel,Obj_XPos,Obj_YPos,Obj_ID,Obj_UpdateFlag,Obj_ValidFlag,Obj_MotionPattern,Obj_Type,Obj_MeasFlag
  Constant : Constant  Value=0  OutDataTypeStr=uint8
  Constant1 : Constant  Value=0  OutDataTypeStr=uint8
  Data Type Conversion : DataTypeConversion  OutDataTypeStr=uint16
  Data Type Conversion{1..5} (5 alike) : DataTypeConversion  OutDataTypeStr=uint8
  <OBJ_36> : Outport
  wires:
  Bus Selector1/10 -> Bus Creator1/10  "<Obj_YPos>"
  Constant1/1 -> Bus Creator/2
  Bus Selector1/8 -> Bus Creator1/8  "<Obj_XVelRel>"
  Bus Selector1/14 -> Data Type Conversion3/1  "<Obj_MotionPattern>"
  Bus Creator1/1 -> <OBJ_36>/1
  Bus Selector1/11 -> Data Type Conversion/1  "<Obj_ID>"
  Bus Selector1/16 -> Data Type Conversion5/1  "<Obj_MeasFlag>"
  Bus Selector1/2 -> Bus Creator1/2  "<Obj_XPos_Stdev>"
  Bus Selector1/6 -> Bus Creator1/6  "<Obj_ExstProb>"
  Bus Selector1/1 -> Bus Creator1/1  "<Obj_ObstacleProb>"
  Bus Selector1/15 -> Data Type Conversion4/1  "<Obj_Type>"
  Constant/1 -> Bus Creator/1
  Bus Selector1/13 -> Data Type Conversion2/1  "<Obj_ValidFlag>"
  Bus Selector1/9 -> Bus Creator1/9  "<Obj_XPos>"
  Bus Selector1/4 -> Bus Creator1/4  "<Obj_XVelRel_Stdev>"
  Bus Selector1/3 -> Bus Creator1/3  "<Obj_YPos_Stdev>"
  Bus Selector1/5 -> Bus Creator1/5  "<Obj_XAccRel>"
  Bus Selector1/7 -> Bus Creator1/7  "<Obj_YVelRel>"
  Bus Selector1/12 -> Data Type Conversion1/1  "<Obj_UpdateFlag>"
  <x74_44_Obj_36>/1 -> Bus Selector1/1
  Bus Creator/1 -> Bus Creator1/17
  Data Type Conversion/1 -> Bus Creator1/11
  Data Type Conversion1/1 -> Bus Creator1/12
  Data Type Conversion2/1 -> Bus Creator1/13
  Data Type Conversion3/1 -> Bus Creator1/14
  Data Type Conversion4/1 -> Bus Creator1/15
  Data Type Conversion5/1 -> Bus Creator1/16

== system fusionAlg/FUSION /FUS_DataAdapter/RadarAdapter/Subsystem29 ==
  <x75_45_Obj_37> : Inport
  Bus Creator : BusCreator  Inputs=2  OutDataTypeStr=Bus: FUS_UINT8_RESERVED_ST
      settings: InheritFromInputs=off
  Bus Creator1 : BusCreator  Inputs=17  OutDataTypeStr=Bus: FUS_RADAR_OBJ_ST  NonVirtualBus=on
      settings: InheritFromInputs=off
  Bus Selector1 : BusSelector  OutputSignals=Obj_ObstacleProb,Obj_XPos_Stdev,Obj_YPos_Stdev,Obj_XVelRel_Stdev,Obj_XAccRel,Obj_ExstProb,Obj_YVelRel,Obj_XVelRel,Obj_XPos,Obj_YPos,Obj_ID,Obj_UpdateFlag,Obj_ValidFlag,Obj_MotionPattern,Obj_Type,Obj_MeasFlag
  Constant : Constant  Value=0  OutDataTypeStr=uint8
  Constant1 : Constant  Value=0  OutDataTypeStr=uint8
  Data Type Conversion : DataTypeConversion  OutDataTypeStr=uint16
  Data Type Conversion{1..5} (5 alike) : DataTypeConversion  OutDataTypeStr=uint8
  <OBJ_37> : Outport
  wires:
  Bus Selector1/10 -> Bus Creator1/10  "<Obj_YPos>"
  Constant1/1 -> Bus Creator/2
  Bus Selector1/8 -> Bus Creator1/8  "<Obj_XVelRel>"
  Bus Selector1/14 -> Data Type Conversion3/1  "<Obj_MotionPattern>"
  Bus Creator1/1 -> <OBJ_37>/1
  Bus Selector1/11 -> Data Type Conversion/1  "<Obj_ID>"
  Bus Selector1/16 -> Data Type Conversion5/1  "<Obj_MeasFlag>"
  Bus Selector1/2 -> Bus Creator1/2  "<Obj_XPos_Stdev>"
  Bus Selector1/6 -> Bus Creator1/6  "<Obj_ExstProb>"
  Bus Selector1/1 -> Bus Creator1/1  "<Obj_ObstacleProb>"
  Bus Selector1/15 -> Data Type Conversion4/1  "<Obj_Type>"
  Constant/1 -> Bus Creator/1
  Bus Selector1/13 -> Data Type Conversion2/1  "<Obj_ValidFlag>"
  Bus Selector1/9 -> Bus Creator1/9  "<Obj_XPos>"
  Bus Selector1/4 -> Bus Creator1/4  "<Obj_XVelRel_Stdev>"
  Bus Selector1/3 -> Bus Creator1/3  "<Obj_YPos_Stdev>"
  Bus Selector1/5 -> Bus Creator1/5  "<Obj_XAccRel>"
  Bus Selector1/7 -> Bus Creator1/7  "<Obj_YVelRel>"
  Bus Selector1/12 -> Data Type Conversion1/1  "<Obj_UpdateFlag>"
  <x75_45_Obj_37>/1 -> Bus Selector1/1
  Bus Creator/1 -> Bus Creator1/17
  Data Type Conversion/1 -> Bus Creator1/11
  Data Type Conversion1/1 -> Bus Creator1/12
  Data Type Conversion2/1 -> Bus Creator1/13
  Data Type Conversion3/1 -> Bus Creator1/14
  Data Type Conversion4/1 -> Bus Creator1/15
  Data Type Conversion5/1 -> Bus Creator1/16

== system fusionAlg/FUSION /FUS_DataAdapter/RadarAdapter/Subsystem3 ==
  <x53_23_Obj_03> : Inport
  Bus Creator : BusCreator  Inputs=2  OutDataTypeStr=Bus: FUS_UINT8_RESERVED_ST
      settings: InheritFromInputs=off
  Bus Creator1 : BusCreator  Inputs=17  OutDataTypeStr=Bus: FUS_RADAR_OBJ_ST  NonVirtualBus=on
      settings: InheritFromInputs=off
  Bus Selector1 : BusSelector  OutputSignals=Obj_ObstacleProb,Obj_XPos_Stdev,Obj_YPos_Stdev,Obj_XVelRel_Stdev,Obj_XAccRel,Obj_ExstProb,Obj_YVelRel,Obj_XVelRel,Obj_XPos,Obj_YPos,Obj_ID,Obj_UpdateFlag,Obj_ValidFlag,Obj_MotionPattern,Obj_Type,Obj_MeasFlag
  Constant : Constant  Value=0  OutDataTypeStr=uint8
  Constant1 : Constant  Value=0  OutDataTypeStr=uint8
  Data Type Conversion : DataTypeConversion  OutDataTypeStr=uint16
  Data Type Conversion{1..5} (5 alike) : DataTypeConversion  OutDataTypeStr=uint8
  <OBJ_03> : Outport
  wires:
  Bus Selector1/10 -> Bus Creator1/10  "<Obj_YPos>"
  Constant1/1 -> Bus Creator/2
  Bus Selector1/8 -> Bus Creator1/8  "<Obj_XVelRel>"
  Bus Selector1/14 -> Data Type Conversion3/1  "<Obj_MotionPattern>"
  Bus Creator1/1 -> <OBJ_03>/1
  Bus Selector1/11 -> Data Type Conversion/1  "<Obj_ID>"
  Bus Selector1/16 -> Data Type Conversion5/1  "<Obj_MeasFlag>"
  Bus Selector1/2 -> Bus Creator1/2  "<Obj_XPos_Stdev>"
  Bus Selector1/6 -> Bus Creator1/6  "<Obj_ExstProb>"
  Bus Selector1/1 -> Bus Creator1/1  "<Obj_ObstacleProb>"
  Bus Selector1/15 -> Data Type Conversion4/1  "<Obj_Type>"
  Constant/1 -> Bus Creator/1
  Bus Selector1/13 -> Data Type Conversion2/1  "<Obj_ValidFlag>"
  Bus Selector1/9 -> Bus Creator1/9  "<Obj_XPos>"
  Bus Selector1/4 -> Bus Creator1/4  "<Obj_XVelRel_Stdev>"
  Bus Selector1/3 -> Bus Creator1/3  "<Obj_YPos_Stdev>"
  Bus Selector1/5 -> Bus Creator1/5  "<Obj_XAccRel>"
  Bus Selector1/7 -> Bus Creator1/7  "<Obj_YVelRel>"
  Bus Selector1/12 -> Data Type Conversion1/1  "<Obj_UpdateFlag>"
  <x53_23_Obj_03>/1 -> Bus Selector1/1
  Bus Creator/1 -> Bus Creator1/17
  Data Type Conversion/1 -> Bus Creator1/11
  Data Type Conversion1/1 -> Bus Creator1/12
  Data Type Conversion2/1 -> Bus Creator1/13
  Data Type Conversion3/1 -> Bus Creator1/14
  Data Type Conversion4/1 -> Bus Creator1/15
  Data Type Conversion5/1 -> Bus Creator1/16

== system fusionAlg/FUSION /FUS_DataAdapter/RadarAdapter/Subsystem32 ==
  <x76_46_Obj_38> : Inport
  Bus Creator : BusCreator  Inputs=2  OutDataTypeStr=Bus: FUS_UINT8_RESERVED_ST
      settings: InheritFromInputs=off
  Bus Creator1 : BusCreator  Inputs=17  OutDataTypeStr=Bus: FUS_RADAR_OBJ_ST  NonVirtualBus=on
      settings: InheritFromInputs=off
  Bus Selector1 : BusSelector  OutputSignals=Obj_ObstacleProb,Obj_XPos_Stdev,Obj_YPos_Stdev,Obj_XVelRel_Stdev,Obj_XAccRel,Obj_ExstProb,Obj_YVelRel,Obj_XVelRel,Obj_XPos,Obj_YPos,Obj_ID,Obj_UpdateFlag,Obj_ValidFlag,Obj_MotionPattern,Obj_Type,Obj_MeasFlag
  Constant : Constant  Value=0  OutDataTypeStr=uint8
  Constant1 : Constant  Value=0  OutDataTypeStr=uint8
  Data Type Conversion : DataTypeConversion  OutDataTypeStr=uint16
  Data Type Conversion{1..5} (5 alike) : DataTypeConversion  OutDataTypeStr=uint8
  <OBJ_38> : Outport
  wires:
  Bus Selector1/10 -> Bus Creator1/10  "<Obj_YPos>"
  Constant1/1 -> Bus Creator/2
  Bus Selector1/8 -> Bus Creator1/8  "<Obj_XVelRel>"
  Bus Selector1/14 -> Data Type Conversion3/1  "<Obj_MotionPattern>"
  Bus Creator1/1 -> <OBJ_38>/1
  Bus Selector1/11 -> Data Type Conversion/1  "<Obj_ID>"
  Bus Selector1/16 -> Data Type Conversion5/1  "<Obj_MeasFlag>"
  Bus Selector1/2 -> Bus Creator1/2  "<Obj_XPos_Stdev>"
  Bus Selector1/6 -> Bus Creator1/6  "<Obj_ExstProb>"
  Bus Selector1/1 -> Bus Creator1/1  "<Obj_ObstacleProb>"
  Bus Selector1/15 -> Data Type Conversion4/1  "<Obj_Type>"
  Constant/1 -> Bus Creator/1
  Bus Selector1/13 -> Data Type Conversion2/1  "<Obj_ValidFlag>"
  Bus Selector1/9 -> Bus Creator1/9  "<Obj_XPos>"
  Bus Selector1/4 -> Bus Creator1/4  "<Obj_XVelRel_Stdev>"
  Bus Selector1/3 -> Bus Creator1/3  "<Obj_YPos_Stdev>"
  Bus Selector1/5 -> Bus Creator1/5  "<Obj_XAccRel>"
  Bus Selector1/7 -> Bus Creator1/7  "<Obj_YVelRel>"
  Bus Selector1/12 -> Data Type Conversion1/1  "<Obj_UpdateFlag>"
  <x76_46_Obj_38>/1 -> Bus Selector1/1
  Bus Creator/1 -> Bus Creator1/17
  Data Type Conversion/1 -> Bus Creator1/11
  Data Type Conversion1/1 -> Bus Creator1/12
  Data Type Conversion2/1 -> Bus Creator1/13
  Data Type Conversion3/1 -> Bus Creator1/14
  Data Type Conversion4/1 -> Bus Creator1/15
  Data Type Conversion5/1 -> Bus Creator1/16

== system fusionAlg/FUSION /FUS_DataAdapter/RadarAdapter/Subsystem33 ==
  <x77_47_Obj_39> : Inport
  Bus Creator : BusCreator  Inputs=2  OutDataTypeStr=Bus: FUS_UINT8_RESERVED_ST
      settings: InheritFromInputs=off
  Bus Creator1 : BusCreator  Inputs=17  OutDataTypeStr=Bus: FUS_RADAR_OBJ_ST  NonVirtualBus=on
      settings: InheritFromInputs=off
  Bus Selector1 : BusSelector  OutputSignals=Obj_ObstacleProb,Obj_XPos_Stdev,Obj_YPos_Stdev,Obj_XVelRel_Stdev,Obj_XAccRel,Obj_ExstProb,Obj_YVelRel,Obj_XVelRel,Obj_XPos,Obj_YPos,Obj_ID,Obj_UpdateFlag,Obj_ValidFlag,Obj_MotionPattern,Obj_Type,Obj_MeasFlag
  Constant : Constant  Value=0  OutDataTypeStr=uint8
  Constant1 : Constant  Value=0  OutDataTypeStr=uint8
  Data Type Conversion : DataTypeConversion  OutDataTypeStr=uint16
  Data Type Conversion{1..5} (5 alike) : DataTypeConversion  OutDataTypeStr=uint8
  <OBJ_39> : Outport
  wires:
  Bus Selector1/10 -> Bus Creator1/10  "<Obj_YPos>"
  Constant1/1 -> Bus Creator/2
  Bus Selector1/8 -> Bus Creator1/8  "<Obj_XVelRel>"
  Bus Selector1/14 -> Data Type Conversion3/1  "<Obj_MotionPattern>"
  Bus Creator1/1 -> <OBJ_39>/1
  Bus Selector1/11 -> Data Type Conversion/1  "<Obj_ID>"
  Bus Selector1/16 -> Data Type Conversion5/1  "<Obj_MeasFlag>"
  Bus Selector1/2 -> Bus Creator1/2  "<Obj_XPos_Stdev>"
  Bus Selector1/6 -> Bus Creator1/6  "<Obj_ExstProb>"
  Bus Selector1/1 -> Bus Creator1/1  "<Obj_ObstacleProb>"
  Bus Selector1/15 -> Data Type Conversion4/1  "<Obj_Type>"
  Constant/1 -> Bus Creator/1
  Bus Selector1/13 -> Data Type Conversion2/1  "<Obj_ValidFlag>"
  Bus Selector1/9 -> Bus Creator1/9  "<Obj_XPos>"
  Bus Selector1/4 -> Bus Creator1/4  "<Obj_XVelRel_Stdev>"
  Bus Selector1/3 -> Bus Creator1/3  "<Obj_YPos_Stdev>"
  Bus Selector1/5 -> Bus Creator1/5  "<Obj_XAccRel>"
  Bus Selector1/7 -> Bus Creator1/7  "<Obj_YVelRel>"
  Bus Selector1/12 -> Data Type Conversion1/1  "<Obj_UpdateFlag>"
  <x77_47_Obj_39>/1 -> Bus Selector1/1
  Bus Creator/1 -> Bus Creator1/17
  Data Type Conversion/1 -> Bus Creator1/11
  Data Type Conversion1/1 -> Bus Creator1/12
  Data Type Conversion2/1 -> Bus Creator1/13
  Data Type Conversion3/1 -> Bus Creator1/14
  Data Type Conversion4/1 -> Bus Creator1/15
  Data Type Conversion5/1 -> Bus Creator1/16

== system fusionAlg/FUSION /FUS_DataAdapter/RadarAdapter/Subsystem36 ==
  <x6A_3A_Obj_26> : Inport
  Bus Creator : BusCreator  Inputs=2  OutDataTypeStr=Bus: FUS_UINT8_RESERVED_ST
      settings: InheritFromInputs=off
  Bus Creator1 : BusCreator  Inputs=17  OutDataTypeStr=Bus: FUS_RADAR_OBJ_ST  NonVirtualBus=on
      settings: InheritFromInputs=off
  Bus Selector1 : BusSelector  OutputSignals=Obj_ObstacleProb,Obj_XPos_Stdev,Obj_YPos_Stdev,Obj_XVelRel_Stdev,Obj_XAccRel,Obj_ExstProb,Obj_YVelRel,Obj_XVelRel,Obj_XPos,Obj_YPos,Obj_ID,Obj_UpdateFlag,Obj_ValidFlag,Obj_MotionPattern,Obj_Type,Obj_MeasFlag
  Constant : Constant  Value=0  OutDataTypeStr=uint8
  Constant1 : Constant  Value=0  OutDataTypeStr=uint8
  Data Type Conversion : DataTypeConversion  OutDataTypeStr=uint16
  Data Type Conversion{1..5} (5 alike) : DataTypeConversion  OutDataTypeStr=uint8
  <OBJ_26> : Outport
  wires:
  Bus Selector1/10 -> Bus Creator1/10  "<Obj_YPos>"
  Constant1/1 -> Bus Creator/2
  Bus Selector1/8 -> Bus Creator1/8  "<Obj_XVelRel>"
  Bus Selector1/14 -> Data Type Conversion3/1  "<Obj_MotionPattern>"
  Bus Creator1/1 -> <OBJ_26>/1
  Bus Selector1/11 -> Data Type Conversion/1  "<Obj_ID>"
  Bus Selector1/16 -> Data Type Conversion5/1  "<Obj_MeasFlag>"
  Bus Selector1/2 -> Bus Creator1/2  "<Obj_XPos_Stdev>"
  Bus Selector1/6 -> Bus Creator1/6  "<Obj_ExstProb>"
  Bus Selector1/1 -> Bus Creator1/1  "<Obj_ObstacleProb>"
  Bus Selector1/15 -> Data Type Conversion4/1  "<Obj_Type>"
  Constant/1 -> Bus Creator/1
  Bus Selector1/13 -> Data Type Conversion2/1  "<Obj_ValidFlag>"
  Bus Selector1/9 -> Bus Creator1/9  "<Obj_XPos>"
  Bus Selector1/4 -> Bus Creator1/4  "<Obj_XVelRel_Stdev>"
  Bus Selector1/3 -> Bus Creator1/3  "<Obj_YPos_Stdev>"
  Bus Selector1/5 -> Bus Creator1/5  "<Obj_XAccRel>"
  Bus Selector1/7 -> Bus Creator1/7  "<Obj_YVelRel>"
  Bus Selector1/12 -> Data Type Conversion1/1  "<Obj_UpdateFlag>"
  <x6A_3A_Obj_26>/1 -> Bus Selector1/1
  Bus Creator/1 -> Bus Creator1/17
  Data Type Conversion/1 -> Bus Creator1/11
  Data Type Conversion1/1 -> Bus Creator1/12
  Data Type Conversion2/1 -> Bus Creator1/13
  Data Type Conversion3/1 -> Bus Creator1/14
  Data Type Conversion4/1 -> Bus Creator1/15
  Data Type Conversion5/1 -> Bus Creator1/16

== system fusionAlg/FUSION /FUS_DataAdapter/RadarAdapter/Subsystem4 ==
  <x54_24_Obj_04> : Inport
  Bus Creator : BusCreator  Inputs=2  OutDataTypeStr=Bus: FUS_UINT8_RESERVED_ST
      settings: InheritFromInputs=off
  Bus Creator1 : BusCreator  Inputs=17  OutDataTypeStr=Bus: FUS_RADAR_OBJ_ST  NonVirtualBus=on
      settings: InheritFromInputs=off
  Bus Selector1 : BusSelector  OutputSignals=Obj_ObstacleProb,Obj_XPos_Stdev,Obj_YPos_Stdev,Obj_XVelRel_Stdev,Obj_XAccRel,Obj_ExstProb,Obj_YVelRel,Obj_XVelRel,Obj_XPos,Obj_YPos,Obj_ID,Obj_UpdateFlag,Obj_ValidFlag,Obj_MotionPattern,Obj_Type,Obj_MeasFlag
  Constant : Constant  Value=0  OutDataTypeStr=uint8
  Constant1 : Constant  Value=0  OutDataTypeStr=uint8
  Data Type Conversion : DataTypeConversion  OutDataTypeStr=uint16
  Data Type Conversion{1..5} (5 alike) : DataTypeConversion  OutDataTypeStr=uint8
  <OBJ_04> : Outport
  wires:
  Bus Selector1/10 -> Bus Creator1/10  "<Obj_YPos>"
  Constant1/1 -> Bus Creator/2
  Bus Selector1/8 -> Bus Creator1/8  "<Obj_XVelRel>"
  Bus Selector1/14 -> Data Type Conversion3/1  "<Obj_MotionPattern>"
  Bus Creator1/1 -> <OBJ_04>/1
  Bus Selector1/11 -> Data Type Conversion/1  "<Obj_ID>"
  Bus Selector1/16 -> Data Type Conversion5/1  "<Obj_MeasFlag>"
  Bus Selector1/2 -> Bus Creator1/2  "<Obj_XPos_Stdev>"
  Bus Selector1/6 -> Bus Creator1/6  "<Obj_ExstProb>"
  Bus Selector1/1 -> Bus Creator1/1  "<Obj_ObstacleProb>"
  Bus Selector1/15 -> Data Type Conversion4/1  "<Obj_Type>"
  Constant/1 -> Bus Creator/1
  Bus Selector1/13 -> Data Type Conversion2/1  "<Obj_ValidFlag>"
  Bus Selector1/9 -> Bus Creator1/9  "<Obj_XPos>"
  Bus Selector1/4 -> Bus Creator1/4  "<Obj_XVelRel_Stdev>"
  Bus Selector1/3 -> Bus Creator1/3  "<Obj_YPos_Stdev>"
  Bus Selector1/5 -> Bus Creator1/5  "<Obj_XAccRel>"
  Bus Selector1/7 -> Bus Creator1/7  "<Obj_YVelRel>"
  Bus Selector1/12 -> Data Type Conversion1/1  "<Obj_UpdateFlag>"
  <x54_24_Obj_04>/1 -> Bus Selector1/1
  Bus Creator/1 -> Bus Creator1/17
  Data Type Conversion/1 -> Bus Creator1/11
  Data Type Conversion1/1 -> Bus Creator1/12
  Data Type Conversion2/1 -> Bus Creator1/13
  Data Type Conversion3/1 -> Bus Creator1/14
  Data Type Conversion4/1 -> Bus Creator1/15
  Data Type Conversion5/1 -> Bus Creator1/16

== system fusionAlg/FUSION /FUS_DataAdapter/RadarAdapter/Subsystem40 ==
  <x80_Status> : Inport
  Bus Creator1 : BusCreator  Inputs=12  OutDataTypeStr=Bus: FUS_RADAR_STATE_ST  NonVirtualBus=on
      settings: InheritFromInputs=off
  Bus Creator2 : BusCreator  Inputs=2  OutDataTypeStr=Bus: FUS_UINT8_RESERVED_ST  NonVirtualBus=on
      settings: InheritFromInputs=off
  Bus Selector1 : BusSelector  OutputSignals=Host_Yaw,HostSpeed,TimeStamp,Status_HWErr,Status_BlkProg,Status_MisAlign,Fail,MeasEnabled,Msg_AliveCounter,Latency,Msg_CheckSum
  Constant : Constant  Value=0  OutDataTypeStr=uint8
  Constant1 : Constant  Value=0  OutDataTypeStr=uint8
  Data Type Conversion : DataTypeConversion  OutDataTypeStr=uint16
  Data Type Conversion{1..8} (8 alike) : DataTypeConversion  OutDataTypeStr=uint8
  <STATUS> : Outport
  wires:
  Bus Selector1/4 -> Data Type Conversion1/1  "<Status_HWErr>"
  Bus Selector1/5 -> Data Type Conversion2/1  "<Status_BlkProg>"
  Bus Selector1/2 -> Bus Creator1/2  "<HostSpeed>"
  Bus Selector1/10 -> Data Type Conversion7/1  "<Latency>"
  Constant/1 -> Bus Creator2/1
  <x80_Status>/1 -> Bus Selector1/1
  Bus Selector1/11 -> Data Type Conversion8/1  "<Msg_CheckSum>"
  Bus Selector1/9 -> Data Type Conversion6/1  "<Msg_AliveCounter>"
  Bus Selector1/1 -> Bus Creator1/1  "<Host_Yaw>"
  Bus Selector1/8 -> Data Type Conversion5/1  "<MeasEnabled>"
  Constant1/1 -> Bus Creator2/2
  Bus Creator2/1 -> Bus Creator1/12
  Data Type Conversion/1 -> Bus Creator1/3
  Bus Creator1/1 -> <STATUS>/1
  Data Type Conversion1/1 -> Bus Creator1/4
  Bus Selector1/3 -> Data Type Conversion/1  "<TimeStamp>"
  Data Type Conversion2/1 -> Bus Creator1/5
  Data Type Conversion3/1 -> Bus Creator1/6
  Bus Selector1/6 -> Data Type Conversion3/1  "<Status_MisAlign>"
  Bus Selector1/7 -> Data Type Conversion4/1  "<Fail>"
  Data Type Conversion4/1 -> Bus Creator1/7
  Data Type Conversion5/1 -> Bus Creator1/8
  Data Type Conversion6/1 -> Bus Creator1/9
  Data Type Conversion7/1 -> Bus Creator1/10
  Data Type Conversion8/1 -> Bus Creator1/11
